simulink model "MG_lossless"  (R2019b)
settings: Solver=ode4  StartTime=0.0  StopTime=TFinal  RelTol=1e-3
undefined symbols (not defined in the file or in its folder): coupling, decay_rate, n, sample_time
libraries: simrfV2util1 x32, simrfV2elements x32, simrfV2_lib x1
settings Model: Creator=tg847  LastModifiedBy=tg847

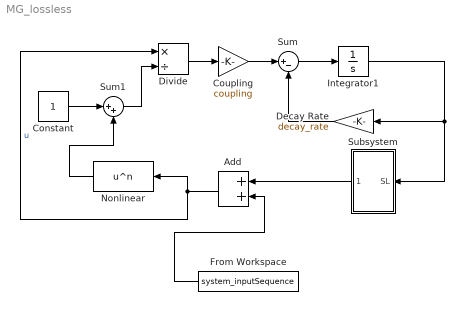
== system MG_lossless ==
  Add : Sum
  Constant : Constant
  Coupling : Gain  Gain=coupling
      mask Display: fprintf("%c", 946)
  "Decay Rate " : Gain  Gain=decay_rate
      mask Display: fprintf("%c", 947)
  Divide : Product  Inputs=*/
  From Workspace : FromWorkspace  VariableName=system_inputSequence  SampleTime=0
  Integrator1 : Integrator  IgnoreLimit=on
  Nonlinear : Fcn  Expr=u^n
  Subsystem : Subsystem
  Sum : Sum  Inputs=|+-
  Sum1 : Sum  Inputs=|++
  wires:
  Coupling/1 -> Sum/1
  Add/1 -> Divide/1, Nonlinear/1  "u"
  "Decay Rate "/1 -> Sum/2
  Subsystem/1(SL1) -> Add/1
  Constant/1 -> Sum1/1
  Divide/1 -> Coupling/1
  From Workspace/1 -> Add/2
  Nonlinear/1 -> Sum1/2
  Sum/1 -> Integrator1/1
  Sum1/1 -> Divide/2
  Integrator1/1 -> "Decay Rate "/1, Subsystem/1(SL)

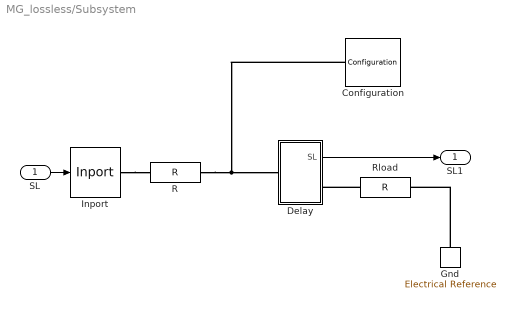
== system MG_lossless/Subsystem ==
  SL : Inport
  Configuration : simrfV2util1/Configuration  AutoFreq=on  Tones=[0] Hz  Harmonics=[1]  NormalizeCarrierPower=on  SolverType=Auto  UseCCode=on  StepSize=0.06/10 s  AddNoise=on  defaultRNG=on  Seed=0  Temperature=290 K  SolverDelFlag=0  AbsTol=1e-6  RelTol=1e-3  MaxIter=10  ErrorEstimationType=2-norm over all variables  EnableInterpFilter=off  HiddenFIRfilterControllerParam=on  SmallSignalApprox=off  AllSimFreqs=on  SimFreqs=[] Hz  SimFreqsInternal=[]  SamplesPerFrame=1
      settings: SourceProductName=RF Blockset  SourceProductBaseCode=RB
  Delay : Subsystem
  Gnd : simrfV2_lib/Elements/Electrical Reference
      settings: SourceProductName=RF Blockset  SourceProductBaseCode=RB  InternalSimscapePortConfiguration="{\"Bottom\":[],\"Left\":[{\"id\":\"V\",\"label\":\"\",\"type\":\"foundation.rf.circuitenvelope\"}],\"Right\":[],\"Top\":[]}"
  Inport : simrfV2util1/Inport  SimulinkInputSignalType=Ideal voltage  CarrierFreq=0 Hz  ZS=0  InternalGrounding=on
      settings: SourceProductName=RF Blockset  SourceProductBaseCode=RB
  R : simrfV2elements/R  classname=resistor  Resistance=135/2 Ohm  AddNoise=off
      settings: SourceProductName=RF Blockset  SourceProductBaseCode=RB
  Rload : simrfV2elements/R  classname=resistor  Resistance=135/2 Ohm  AddNoise=off
      settings: SourceProductName=RF Blockset  SourceProductBaseCode=RB
  SL1 : Outport
  wires:
  SL/1 -> Inport/1
  Delay/1(SL) -> SL1/1
  connections:
  Inport/RConn1 -- R/LConn1
  R/RConn1 -- Configuration/LConn1 -- Delay/LConn1
  Gnd/LConn1 -- Rload/LConn1
  Rload/RConn1 -- Delay/RConn1

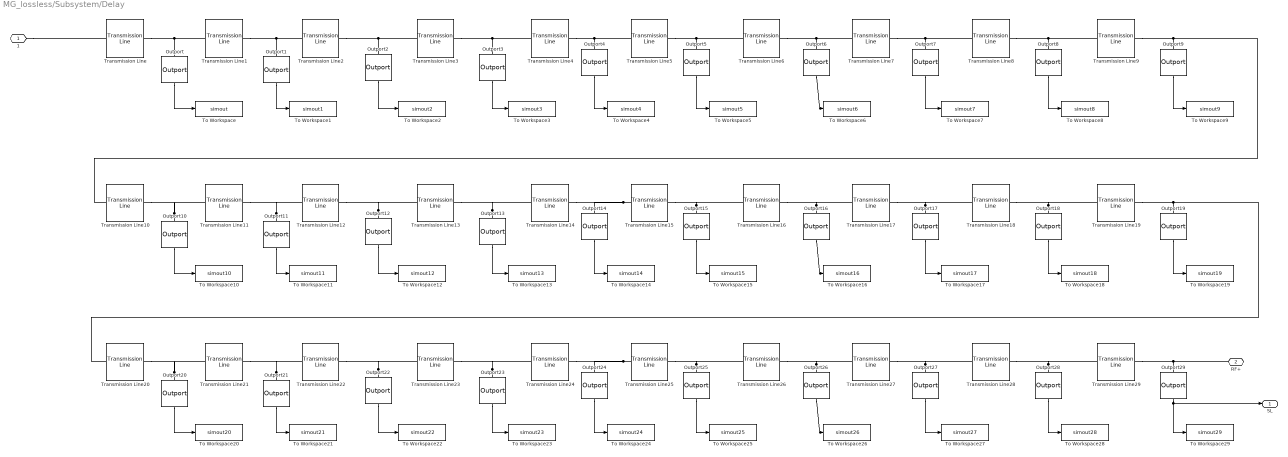
== system MG_lossless/Subsystem/Delay ==
  Outport{,1..29} (30 alike) : simrfV2util1/Outport  SensorType=Ideal voltage  OutputFormat=Real Passband  CarrierFreq=0 Hz  ZL=Inf  InternalGrounding=on  StepSize=1e-06 s  AutoStep=on
      settings: SourceProductName=RF Blockset  SourceProductBaseCode=RB
  To Workspace : ToWorkspace  VariableName=simout  SampleTime=sample_time
  To Workspace1 : ToWorkspace  VariableName=simout1  SampleTime=sample_time
  To Workspace10 : ToWorkspace  VariableName=simout10  SampleTime=sample_time
  To Workspace11 : ToWorkspace  VariableName=simout11  SampleTime=sample_time
  To Workspace12 : ToWorkspace  VariableName=simout12  SampleTime=sample_time
  To Workspace13 : ToWorkspace  VariableName=simout13  SampleTime=sample_time
  To Workspace14 : ToWorkspace  VariableName=simout14  SampleTime=sample_time
  To Workspace15 : ToWorkspace  VariableName=simout15  SampleTime=sample_time
  To Workspace16 : ToWorkspace  VariableName=simout16  SampleTime=sample_time
  To Workspace17 : ToWorkspace  VariableName=simout17  SampleTime=sample_time
  To Workspace18 : ToWorkspace  VariableName=simout18  SampleTime=sample_time
  To Workspace19 : ToWorkspace  VariableName=simout19  SampleTime=sample_time
  To Workspace2 : ToWorkspace  VariableName=simout2  SampleTime=sample_time
  To Workspace20 : ToWorkspace  VariableName=simout20  SampleTime=sample_time
  To Workspace21 : ToWorkspace  VariableName=simout21  SampleTime=sample_time
  To Workspace22 : ToWorkspace  VariableName=simout22  SampleTime=sample_time
  To Workspace23 : ToWorkspace  VariableName=simout23  SampleTime=sample_time
  To Workspace24 : ToWorkspace  VariableName=simout24  SampleTime=sample_time
  To Workspace25 : ToWorkspace  VariableName=simout25  SampleTime=sample_time
  To Workspace26 : ToWorkspace  VariableName=simout26  SampleTime=sample_time
  To Workspace27 : ToWorkspace  VariableName=simout27  SampleTime=sample_time
  To Workspace28 : ToWorkspace  VariableName=simout28  SampleTime=sample_time
  To Workspace29 : ToWorkspace  VariableName=simout29  SampleTime=sample_time
  To Workspace3 : ToWorkspace  VariableName=simout3  SampleTime=sample_time
  To Workspace4 : ToWorkspace  VariableName=simout4  SampleTime=sample_time
  To Workspace5 : ToWorkspace  VariableName=simout5  SampleTime=sample_time
  To Workspace6 : ToWorkspace  VariableName=simout6  SampleTime=sample_time
  To Workspace7 : ToWorkspace  VariableName=simout7  SampleTime=sample_time
  To Workspace8 : ToWorkspace  VariableName=simout8  SampleTime=sample_time
  To Workspace9 : ToWorkspace  VariableName=simout9  SampleTime=sample_time
  Transmission Line{,1..29} (30 alike) : simrfV2elements/Transmission Line  classname=xline  Model_type=Delay-based and lossless  Parameterization=By inductance and capacitance  TransDelay=theta s  CharImped=135 Ohm  Resistance=10 Ohm/m  Inductance=235e-9 H/m  Capacitance=94e-12 F/m  Conductance=5e-6 S/m  LineLength=1 m  NumSegments=1  InternalGrounding=on  OuterRadius=2.57 mm  InnerRadius=0.725 mm  MuR=1  EpsilonR=2.2  LossTangent=0  SigmaCond=inf S/m  StubMode=Not a stub  Termination=Open  ConductorWidth=0.6 mm  SlotWidth=0.2 mm  Height=0.635 mm  Thickness=5 um  SWidth=0.6 mm  Radius=0.67 mm  Separation=1.62 mm  PWidth=5 mm  PSeparation=1 mm  PV=299792458  Loss=1  SourceFreq=User-specified  PlotFreq=[1e9:1e6:3e9] Hz  PlotType=X-Y plane  YParam1=S11  YFormat1=Magnitude (decibels)  YParam2=S22  YFormat2=Magnitude (decibels)  YOption=Linear  XOption=Linear  FitOpt=Share all poles  FitTol=-40  SparamRepresentation=Frequency domain  Freq=1e9 Hz  Interp_type=Linear  AutoImpulseLength=off  ImpulseLength=0 s  MagModeling=off
      settings: SourceProductName=RF Blockset  SourceProductBaseCode=RB
  1 : PMIOPort  Side=Left
  RF+ : PMIOPort  Port=2  Side=Right
  SL : Outport
  wires:
  Outport5/1 -> To Workspace5/1
  Outport3/1 -> To Workspace3/1
  Outport2/1 -> To Workspace2/1
  Outport7/1 -> To Workspace7/1
  Outport9/1 -> To Workspace9/1
  Outport4/1 -> To Workspace4/1
  Outport1/1 -> To Workspace1/1
  Outport6/1 -> To Workspace6/1
  Outport/1 -> To Workspace/1
  Outport8/1 -> To Workspace8/1
  Outport11/1 -> To Workspace11/1
  Outport14/1 -> To Workspace14/1
  Outport13/1 -> To Workspace13/1
  Outport18/1 -> To Workspace18/1
  Outport15/1 -> To Workspace15/1
  Outport19/1 -> To Workspace19/1
  Outport16/1 -> To Workspace16/1
  Outport12/1 -> To Workspace12/1
  Outport17/1 -> To Workspace17/1
  Outport10/1 -> To Workspace10/1
  Outport21/1 -> To Workspace21/1
  Outport24/1 -> To Workspace24/1
  Outport23/1 -> To Workspace23/1
  Outport28/1 -> To Workspace28/1
  Outport25/1 -> To Workspace25/1
  Outport29/1 -> To Workspace29/1, SL/1
  Outport26/1 -> To Workspace26/1
  Outport22/1 -> To Workspace22/1
  Outport27/1 -> To Workspace27/1
  Outport20/1 -> To Workspace20/1
  connections:
  Transmission Line5/RConn1 -- Transmission Line6/LConn1 -- Outport5/LConn1
  1/RConn1 -- Transmission Line/LConn1
  Transmission Line/RConn1 -- Transmission Line1/LConn1 -- Outport/LConn1
  Transmission Line2/RConn1 -- Transmission Line3/LConn1 -- Outport2/LConn1
  Transmission Line4/RConn1 -- Outport4/LConn1 -- Transmission Line5/LConn1
  Transmission Line9/RConn1 -- Outport9/LConn1 -- Transmission Line10/LConn1
  Transmission Line8/RConn1 -- Transmission Line9/LConn1 -- Outport8/LConn1
  Transmission Line3/RConn1 -- Transmission Line4/LConn1 -- Outport3/LConn1
  Transmission Line6/RConn1 -- Transmission Line7/LConn1 -- Outport6/LConn1
  Transmission Line1/RConn1 -- Transmission Line2/LConn1 -- Outport1/LConn1
  Transmission Line7/RConn1 -- Transmission Line8/LConn1 -- Outport7/LConn1
  Transmission Line15/LConn1 -- Outport14/LConn1 -- Transmission Line14/RConn1
  Outport18/LConn1 -- Transmission Line18/RConn1 -- Transmission Line19/LConn1
  Outport15/LConn1 -- Transmission Line15/RConn1 -- Transmission Line16/LConn1
  Outport16/LConn1 -- Transmission Line16/RConn1 -- Transmission Line17/LConn1
  Outport17/LConn1 -- Transmission Line17/RConn1 -- Transmission Line18/LConn1
  Outport12/LConn1 -- Transmission Line12/RConn1 -- Transmission Line13/LConn1
  Outport13/LConn1 -- Transmission Line14/LConn1 -- Transmission Line13/RConn1
  Outport11/LConn1 -- Transmission Line11/RConn1 -- Transmission Line12/LConn1
  Outport10/LConn1 -- Transmission Line10/RConn1 -- Transmission Line11/LConn1
  Transmission Line19/RConn1 -- Transmission Line20/LConn1 -- Outport19/LConn1
  Transmission Line25/LConn1 -- Outport24/LConn1 -- Transmission Line24/RConn1
  Outport28/LConn1 -- Transmission Line28/RConn1 -- Transmission Line29/LConn1
  Outport25/LConn1 -- Transmission Line25/RConn1 -- Transmission Line26/LConn1
  Outport26/LConn1 -- Transmission Line26/RConn1 -- Transmission Line27/LConn1
  Outport27/LConn1 -- Transmission Line27/RConn1 -- Transmission Line28/LConn1
  Outport22/LConn1 -- Transmission Line22/RConn1 -- Transmission Line23/LConn1
  Outport23/LConn1 -- Transmission Line24/LConn1 -- Transmission Line23/RConn1
  Outport21/LConn1 -- Transmission Line21/RConn1 -- Transmission Line22/LConn1
  Outport20/LConn1 -- Transmission Line20/RConn1 -- Transmission Line21/LConn1
  Transmission Line29/RConn1 -- Outport29/LConn1 -- RF+/RConn1
